simulink model "numerique"  (R2017a)
settings: Solver=FixedStepDiscrete  StartTime=0.0  StopTime=6  RelTol=1e-3  EnableMultiTasking=on
values from neighbouring files (symbols this model uses):
  gainCapteur = 12./max(abs(SortieCapteur(:,2)))    [problematiqueM.m]
libraries: commutil2 x3, dspswit3 x2, dsparch4 x2, commsrccod2 x2, commfilt2 x2, dspsrcs4 x1, simulink_extras x1, dspsigops x1
settings Model: Creator=dufd2703  LastModifiedBy=Guacamole
settings OptimizationCC: LifeSpan=inf
settings DebuggingCC: SFUnexpectedBacktrackingDiag=warning  SFNoUnconditionalDefaultTransitionDiag=warning  SFExecutionAtInitializationDiag=none
settings GRTTargetCC: TargetLangStandard=C89/C90 (ANSI)  GeneratePreprocessorConditionals=Disable all
settings ConfigComp: CovMetricSettings=dw  CovHtmlReporting=on  CovSaveCumulativeToWorkspaceVar=on  CovSaveSingleToWorkspaceVar=on  CovExternalEMLEnable=off

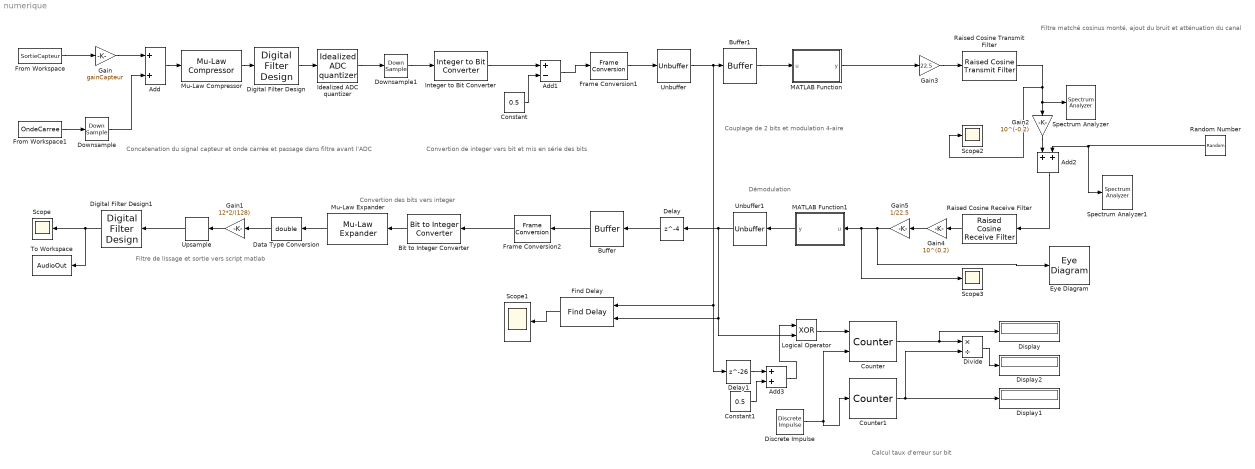
== system numerique ==
  note: Calcul taux d'erreur sur bit
  note: Filtre de lissage et sortie
      | vers script matlab
  note: Convertion des bits vers integer
  note: Démodulation
  note: Filtre matché cosinus monté, ajout du bruit
      | et atténuation du canal
  note: Couplage de 2 bits et modulation 4-aire
  note: Convertion de integer vers bit et mis en série des bits
  note: Concatenation du signal capteur et onde carrée
      | et passage dans filtre avant l'ADC
  Add : Sum
  Add1 : Sum  Inputs=+-
  Add2 : Sum
  Add3 : Sum
  Bit to Integer Converter : commutil2/Bit to Integer Converter  nbits=10  bitOrder=MSB first  signedOutputValues=Signed  outDtype=Inherit via internal rule  outDtypeSigned=Inherit via internal rule
  Buffer : Buffer  N=10
  Buffer1 : Buffer  N=2
  Constant : Constant  Value=0.5
  Constant1 : Constant  Value=0.5
  Counter : dspswit3/Counter  Direction=Up  CountEvent=Rising edge  CounterSize=User defined  MaxCount=100000000  InitialCount=0  Output=Count  HitValue=32  ResetInput=on  SamplesPerFrame=1  Ts=1  CntDtype=double  HitDtype=Logical
  Counter1 : dspswit3/Counter  Direction=Up  CountEvent=Free running  CounterSize=User defined  MaxCount=100000000  InitialCount=0  Output=Count  HitValue=32  ResetInput=on  SamplesPerFrame=1  Ts=1/80000  CntDtype=double  HitDtype=Logical
  Data Type Conversion : DataTypeConversion  OutDataTypeStr=double
  Delay : Delay  DelayLength=4  InitialCondition=0  InputProcessing=Columns as channels (frame based)
  Delay1 : Delay  DelayLength=26  InitialCondition=0
  Digital Filter Design : dsparch4/Digital Filter Design  mwdsp_browser_bugfix_var=off
  Digital Filter Design1 : dsparch4/Digital Filter Design  mwdsp_browser_bugfix_var=off
  Discrete Impulse : dspsrcs4/Discrete  Impulse  Delay=14  SampleTime=1/80000  FrameSample=1  OutputFrames=off  dataType=double  isSigned=on  wordLen=16  udDataType=sfix(16)  fracBitsMode=Best precision  numFracBits=15  OutDataTypeStr=double  LastOutDataTypeStr=double
  Display : Display
  Display1 : Display
  Display2 : Display
  Divide : Product  Inputs=*/
  Downsample : DownSample  N=3  RateOptions=Allow multirate processing
  Downsample1 : DownSample  RateOptions=Allow multirate processing
  Eye Diagram : EyeDiagram
  Find Delay : commutil2/Find Delay  corrLength=200  chgSigOP=off  stopUpdate=off  numConstDelay=10
      settings: SourceProductName=Communications System Toolbox  SourceProductBaseCode=CM
  Frame Conversion1 : FrameConversion  InheritSamplingMode=off
  Frame Conversion2 : FrameConversion  InheritSamplingMode=off  OutFrame=Sample-based
  From Workspace : FromWorkspace  VariableName=SortieCapteur  SampleTime=1/16000  Interpolate=off  OutputAfterFinalValue=Setting to zero
  From Workspace1 : FromWorkspace  VariableName=OndeCarree  SampleTime=1/48000  Interpolate=off  OutputAfterFinalValue=Setting to zero
  Gain : Gain  Gain=gainCapteur
  Gain1 : Gain  Gain=12*2/(128)
  Gain2 : Gain  Gain=10^(-0.2)
  Gain3 : Gain  Gain=22.5
  Gain4 : Gain  Gain=10^(0.2)
  Gain5 : Gain  Gain=1/22.5
  Idealized ADC quantizer : simulink_extras/Additional Discrete/Idealized ADC quantizer  NumberOfConverterBits=10  Vmin=-12  Vmax=12  OutputDataType=double  OutputNegativeValues=on
      settings: SourceProductName=Simulink
  Integer to Bit Converter : commutil2/Integer to Bit Converter  nbits=10  signedInputValues=Signed  bitOrder=MSB first  outDtype=Inherit via internal rule
  Logical Operator : Logic  Operator=XOR  AllPortsSameDT=off  OutDataTypeStr=boolean
  MATLAB Function : MATLAB Function  TreatAsAtomicUnit=on
  MATLAB Function1 : MATLAB Function  TreatAsAtomicUnit=on
  Mu-Law Compressor : commsrccod2/Mu-Law Compressor  mu=200  V=14
      settings: SourceProductName=Communications System Toolbox  SourceProductBaseCode=CM
  Mu-Law Expander : commsrccod2/Mu-Law Expander  mu=200  V=1050
      settings: SourceProductName=Communications System Toolbox  SourceProductBaseCode=CM
  Raised Cosine Receive Filter : commfilt2/Raised Cosine Receive Filter  filtType=Square root  R=0.2  filtSpan=10  N=20  downFactor=20  downOffset=0  filterGain=1  RateOptions=Allow multirate processing  framing=Mute  checkCoeff=off  variableName=rcRxFilt  currentFiltSpan=10  D=(10)/2  inputOffset=0  sampMode=Mute  saveAsFlag=0  rateMode=Downsampling  checkGain=Normalized  launchFVT=on  roundingMode=Floor  overflowMode=off  coeffDataTypeStr=Inherit: Same word length as input  coeffMin=[]  coeffMax=[]  coeffLastDataTypeStr=Inherit: Same word length as input  accumDataTypeStr=Inherit: Same as product output  accumLastDataTypeStr=Inherit: Same as product output  outputDataTypeStr=Inherit: Same as accumulator  outputMin=[]  outputMax=[]  outputLastDataTypeStr=Inherit: Same as accumulator
  Raised Cosine Transmit Filter : commfilt2/Raised Cosine Transmit Filter  filtType=Square root  R=0.2  filtSpan=10  N=20  filterGain=1  RateOptions=Allow multirate processing  framing=Mute  checkCoeff=off  variableName=rcTxFilt  checkGain=Normalized  sampMode=Mute  saveAsFlag=0  currentFiltSpan=10  D=(10)/2  launchFVT=on  roundingMode=Floor  overflowMode=off  coeffDataTypeStr=Inherit: Same word length as input  coeffMin=[]  coeffMax=[]  coeffLastDataTypeStr=Inherit: Same word length as input  outputDataTypeStr=Inherit: Same as accumulator  outputMin=[]  outputMax=[]  outputLastDataTypeStr=Inherit: Same as accumulator
  Random Number : RandomNumber  Variance=800000*0.000002  SampleTime=1/(800000)
  Scope{,1..3} (4 alike) : Scope
  Spectrum Analyzer : SpectrumAnalyzer
  Spectrum Analyzer1 : SpectrumAnalyzer
  To Workspace : ToWorkspace  VariableName=AudioOut  SampleTime=-1
      settings: Save2DSignal=2-D array (concatenate along first dimension)
  Unbuffer : Unbuffer
  Unbuffer1 : Unbuffer
  Upsample : dspsigops/Upsample  N=2  phase=0  RateOptions=Allow multirate processing  ic=0  mode=Unused parameter value
  wires:
  From Workspace/1 -> Gain/1
  Gain/1 -> Add/1
  Add/1 -> Mu-Law Compressor/1
  Downsample/1 -> Add/2
  From Workspace1/1 -> Downsample/1
  Data Type Conversion/1 -> Gain1/1
  Gain1/1 -> Upsample/1
  Downsample1/1 -> Integer to Bit Converter/1
  Bit to Integer Converter/1 -> Mu-Law Expander/1
  Frame Conversion1/1 -> Unbuffer/1
  Integer to Bit Converter/1 -> Add1/1
  Constant/1 -> Add1/2
  Buffer/1 -> Frame Conversion2/1
  Frame Conversion2/1 -> Bit to Integer Converter/1
  Digital Filter Design1/1 -> To Workspace/1, Scope/1
  Find Delay/1 -> Scope1/1
  Unbuffer1/1 -> Delay/1, Logical Operator/2, Find Delay/2
  Delay/1 -> Buffer/1
  Unbuffer/1 -> Buffer1/1, Delay1/1, Find Delay/1
  Random Number/1 -> Add2/2, Spectrum Analyzer1/1
  Add1/1 -> Frame Conversion1/1
  Buffer1/1 -> MATLAB Function/1(u)
  MATLAB Function1/1(y) -> Unbuffer1/1
  Add2/1 -> Raised Cosine Receive Filter/1
  Raised Cosine Receive Filter/1 -> Gain4/1
  Gain4/1 -> Gain5/1
  Logical Operator/1 -> Counter/1
  Discrete Impulse/1 -> Counter1/1, Counter/2
  Counter1/1 -> Divide/2, Display1/1
  Counter/1 -> Display/1, Divide/1
  Divide/1 -> Display2/1
  Delay1/1 -> Add3/1
  Constant1/1 -> Add3/2
  Add3/1 -> Logical Operator/1
  MATLAB Function/1(y) -> Gain3/1
  Gain5/1 -> Eye Diagram/1, Scope3/1, MATLAB Function1/1(u)
  Gain3/1 -> Raised Cosine Transmit Filter/1
  Raised Cosine Transmit Filter/1 -> Scope2/1, Spectrum Analyzer/1, Gain2/1
  Idealized ADC quantizer/1 -> Downsample1/1
  Upsample/1 -> Digital Filter Design1/1
  Digital Filter Design/1 -> Idealized ADC quantizer/1
  Mu-Law Compressor/1 -> Digital Filter Design/1
  Mu-Law Expander/1 -> Data Type Conversion/1
  Gain2/1 -> Add2/1

== matlab function numerique/MATLAB Function1 ==
  data: u input; y output
function y = fcn(u)

y = [0;0];
if u > 2/3
    y = [1;0];
end
if u > 0 && u <= 2/3
    y = [1;1];
end
if u <= 0 && u > -2/3 
    y = [0;1];
end
if u <= -2/3
    y = [0;0];
end

== matlab function numerique/MATLAB Function ==
  data: u input; y output
function y = fcn(u)

u = u > 0;
y = 0;
if u == [1;0]
    y = 1;
end
if u == [1;1]
    y = 1/3;
end
if u == [0;1]
    y = -1/3;
end
if u == [0;0]
    y = -1;
end
